simulink model "Optimal_lqr"  (R2018b)
settings: Solver=VariableStepAuto  StartTime=0.0  StopTime=10  RelTol=1e-3
InitFcn:
  | % NOTE: If using VoltPAQ-X1, make sure both Gain switches are set to 3.
  | K_AMP = 3;
  | % Maximum Output Voltage (V): YAW limited to 15 V. PITCH limited to 24 V.
  | VMAX_AMP_P = 24;
  | VMAX_AMP_Y = 15;
  | % Initial Angle of Pitch (rad)
  | theta_0 = -40.5*pi/180;
  | 
  | g = 9.81;
  | 
  | % Pitch and Yaw Motor Armature Resistance (Ohm)
  | R_m_p = 0.83;
  | R_m_y = 1.60;
  | 
  | % Pitch and Yaw Motor Current-Torque Constant (N.m/A)
  | K_t_p = 0.0182;
  | K_t_y = 0.0109;
  | 
  | % Pitch and Yaw Motor Voltage-Torque Constant (N.m/V)
  | K_yp = K_t_p / R_m_p;
  | K_py = K_t_y / R_m_y;
  | 
  | % Pitch and Yaw Viscous Damping Constant (N.m.s/rad)
  | B_p = 0.8;  % tuned while running simulation and experiment in parallel
  | B_y = 0.318; % identified as described in manual
  | 
  | % Mass of the Helicopter (kg)
  | m_heli = 1.3872;
  | 
  | % Mass of the Helicopter with Yoke (kg)
  | m_heli_case = 1.421;
  | 
  | % Distance from Pitch Pivot to Pitch/Front Motor and Yaw/Back Motor(m)
  | r_p = 7.75*0.0254;
  | r_y = (6+5/8)*0.0254;
  | 
  | % Pitch and Yaw Propeller Force-Thrust Constant found Experimentally (N/V)
  | K_f_p = 5*0.2074;
  | K_f_y = 3*0.1426;
  | 
  | % Pitch and Yaw Propeller Torque-Thrust Constant found Experimentally (N.m/V)
  | K_pp = K_f_p * r_p;
  | K_yy = K_f_y * r_y;
  | 
  | % Mass of Pitch/Front Motor and Yaw/Back Motor (kg)
  | m_motor_p = 0.292;
  | m_motor_y = 0.128;
  | 
  | % Mass of Pitch/Front and Yaw/Back Guard + Propeller(kg)
  | m_shield = 0.143 + 0.024;
  | 
  | % Total Mass of Pitch and Yaw Motor/Shield Assemblies (kg)
  | m_props = ( m_motor_p + m_motor_y + 2 * m_shield );
  | 
  | % Mass of Helicopter Body moving about Pitch Axis (kg)
  | m_body_p = m_heli - m_props;
  | 
  | % Mass of Helicopter Body moving about Yaw Axis (kg)
  | m_body_y = m_heli_case - m_props;
  | 
  | % Mass of Metal Shaft Moving about Yaw Axis (kg)
  | m_shaft = 0.151;
  | 
  | % Total Length of Helicopter Body (m)
  | L_body = 19*0.0254;
  | 
  | % Helicopter Center of Mass from Pivot along Pitch Axis (m)
  | l_cm = ( (m_motor_p + m_shield ) * r_p +  (m_motor_y + m_shield ) * r_y ) / ( m_props ) ;
  | 
  | % Length of Metal Shaft Moving about Yaw Axis through slip ring (m)
  | L_shaft = 11 * 0.0254;
  | 
  | % Pitch and Yaw Motor Rotor Moment of Inertia (kg.m^2)
  | J_m_p = 1.91e-6; %1.7070e-5;
  | J_m_y = 1.374e-4; %1.4471e-5;
  | 
  | % Moment of Inertia of Helicopter Body about its CM (kg.m^2)
  | J_body_p = m_body_p * L_body^2 / 12;
  | J_body_y = m_body_y * L_body^2 / 12;
  | 
  | % Moment of Inertia of Metal Shaft about Yaw Axis (kg.m^2)
  | J_shaft = m_shaft * L_shaft^2 / 3; %;0.0851;
  | 
  | % Moment of Inertia of Pitch Motor + Guard Assembly about Pivot (kg.m^2)
  | J_p = ( m_motor_p + m_shield ) * r_p^2;
  | 
  | % Moment of Inertia of Yaw Motor + Guard Assembly about Pivot (kg.m^2)
  | J_y = ( m_motor_y + m_shield ) * r_y^2;
  | 
  | % Equivalent Moment of Inertia about Pitch and Yaw Axis (kg.m^2)
  | J_eq_p = J_m_p + J_body_p + J_p + J_y;
  | J_eq_y = J_m_y + J_body_y + J_p + J_y + J_shaft;
  | 
  | 
  | %BESSEL wn=4
  | Kbes=[     68.5119  -25.1203    5.3421   -3.6881
  |    63.1652  188.4894    0.7783   19.4789];
  | 
  | xd=-20;
libraries: simulink x1
settings Model: Creator=rezan  LastModifiedBy=rezan
settings DataIOCC: ReturnWorkspaceOutputs=on
settings DebuggingCC: UnconnectedInputMsg=none  UnconnectedOutputMsg=none  UnconnectedLineMsg=none  SFMachineParentedDataDiag=error

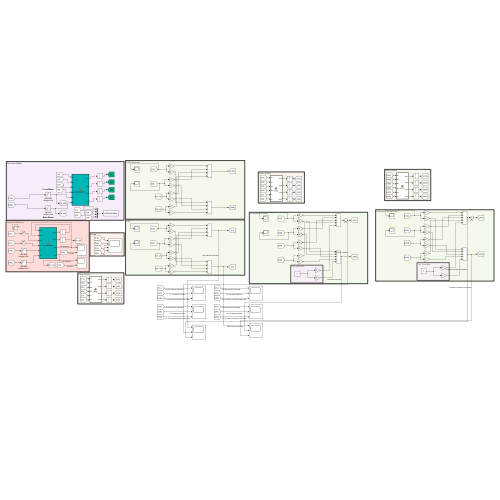
[thumbnail: Simulink's stored preview of the top-level diagram]
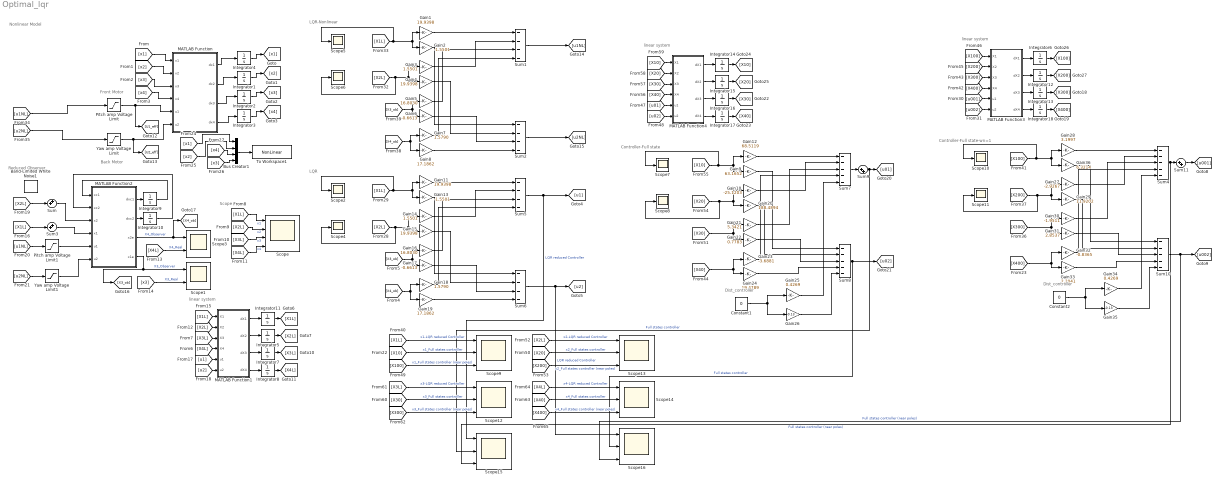
== system Optimal_lqr ==
  note: linear system
  note: Front Motor
  note: Back Motor
  note: Nonlinear Model
  note: Scope
  note: LQR
  note: Reduced Observer
  note: LQR-Nonlinear
  note: Dist_controller
  note: Controller-Full state
  note: linear system
  note: Dist_controller
  note: Controller-Full state-wn=1
  note: linear system
  Band-Limited White Noise1 : simulink/Sources/Band-Limited White Noise  Cov=[0.01]  Ts=0.1  seed=[23341]
  Bus Creator1 : BusCreator  Inputs=4
  Constant1 : Constant  Value=0
  Constant2 : Constant  Value=0
  Gain{1,4,11,15} (4 alike) : Gain  Gain=19.9398
  Gain10 : Gain  Gain=-25.1203
  Gain12 : Gain  Gain=68.5119
  Gain13 : Gain  Gain=-1.5501
  Gain14 : Gain  Gain=1.5501
  Gain16 : Gain  Gain=16.8030
  Gain17 : Gain  Gain=-0.6613
  Gain18 : Gain  Gain=1.5790
  Gain19 : Gain  Gain=17.1862
  Gain2 : Gain  Gain=-1.5501
  Gain20 : Gain  Gain=188.4894
  Gain21 : Gain  Gain=5.3421
  Gain22 : Gain  Gain=0.7783
  Gain23 : Gain  Gain=-3.6881
  Gain24 : Gain  Gain=19.4789
  Gain25 : Gain  Gain=0.4269
  Gain26 : Gain  Gain=-0.13
  Gain27 : Gain  Gain=-2.9267
  Gain28 : Gain  Gain=3.1997
  Gain29 : Gain  Gain=11.9202
  Gain3 : Gain  Gain=1.5501
  Gain30 : Gain  Gain=-1.9511
  Gain31 : Gain  Gain=2.8537
  Gain32 : Gain  Gain=-0.8365
  Gain33 : Gain  Gain=2.3041
  Gain34 : Gain  Gain=0.4269
  Gain35 : Gain  Gain=-0.13
  Gain36 : Gain  Gain=6.3214
  Gain5 : Gain  Gain=16.8030
  Gain6 : Gain  Gain=-0.6613
  Gain7 : Gain  Gain=1.5790
  Gain8 : Gain  Gain=17.1862
  Gain9 : Gain  Gain=63.1652
  Integrator{1,5,12,15} (4 alike) : Integrator  InitialCondition=10*pi/180
  Integrator{2..3,8..10,17..18} (7 alike) : Integrator
  Integrator{4,6,11,14} (4 alike) : Integrator  UpperSaturationLimit=40.5*pi/180  LowerSaturationLimit=-40.5*pi/180
  Integrator13 : Integrator  InitialCondition=10
  Integrator16 : Integrator  InitialCondition=10
  Integrator7 : Integrator  InitialCondition=10
  MATLAB Function : MATLAB Function  TreatAsAtomicUnit=on
  MATLAB Function1 : MATLAB Function  TreatAsAtomicUnit=on
  MATLAB Function2 : MATLAB Function  TreatAsAtomicUnit=on
  MATLAB Function3 : MATLAB Function  TreatAsAtomicUnit=on
  MATLAB Function4 : MATLAB Function  TreatAsAtomicUnit=on
  Pitch amp Voltage Limit : Saturate  UpperLimit=VMAX_AMP_P  LowerLimit=- VMAX_AMP_P
  Pitch amp Voltage Limit1 : Saturate  UpperLimit=VMAX_AMP_P  LowerLimit=- VMAX_AMP_P
  Scope : Scope  NumInputPorts=4
  Scope1 : Scope  NumInputPorts=2
  Scope{2,4..8,10..11} (8 alike) : Scope
  Scope{9,12..16} (6 alike) : Scope  NumInputPorts=3
  Scope3 : Scope  NumInputPorts=2
  Sum : Sum  Inputs=++|
  Sum{1..2,5..6} (4 alike) : Sum  Inputs=----
  Sum{4,7..8,10} (4 alike) : Sum  Inputs=-----
  Sum11 : Sum  Inputs=|++
  Sum3 : Sum  Inputs=++|
  Sum9 : Sum  Inputs=|++
  To Workspace1 : ToWorkspace  VariableName=NonLinear  SampleTime=-1
  Yaw amp Voltage Limit : Saturate  UpperLimit=VMAX_AMP_Y  LowerLimit=- VMAX_AMP_Y
  Yaw amp Voltage Limit1 : Saturate  UpperLimit=VMAX_AMP_Y  LowerLimit=- VMAX_AMP_Y
  wires:
  MATLAB Function/2(dx2) -> Integrator1/1
  [X1L] -> Gain13/1, Gain11/1, Scope2/1
  Gain11/1 -> Sum5/1
  Yaw amp Voltage Limit1/1 -> MATLAB Function2/6(u2)
  [X1L] -> Scope/1  "x1"
  Integrator2/1 -> [x3]
  [X2L] -> Gain15/1, Gain14/1, Scope4/1
  Integrator4/1 -> [x1]
  MATLAB Function/3(dx3) -> Integrator2/1
  MATLAB Function/1(dx1) -> Integrator4/1
  [x1] -> MATLAB Function/1(x1)
  [x1] -> Bus Creator1/1
  [x2] -> Bus Creator1/2
  [x3] -> MATLAB Function/3(x3)
  [x4] -> MATLAB Function/4(x4)
  [x3] -> Bus Creator1/4
  Integrator3/1 -> [x4]
  Integrator9/1 -> MATLAB Function2/1(xc1)
  Gain16/1 -> Sum5/3
  Bus Creator1/1 -> To Workspace1/1
  Integrator1/1 -> [x2]
  [X4L] -> Scope3/2  "X4_Real"
  MATLAB Function2/1(dxc1) -> Integrator9/1
  [u2NL] -> Yaw amp Voltage Limit1/1
  [x3] -> Scope1/2  "X3_Real"
  Yaw amp Voltage Limit/1 -> [U2_eff], MATLAB Function/6(u2)
  MATLAB Function2/4(x1e) -> Scope1/1, [X3_ob]  "X3_Observer"
  Pitch amp Voltage Limit1/1 -> MATLAB Function2/5(u1)
  Gain18/1 -> Sum5/4
  Gain17/1 -> Sum6/3
  MATLAB Function2/3(x2e) -> [X4_ob], Scope3/1  "X4_Observer"
  Integrator10/1 -> MATLAB Function2/2(xc2)
  [u1NL] -> Pitch amp Voltage Limit1/1
  Gain19/1 -> Sum6/4
  MATLAB Function2/2(dxc2) -> Integrator10/1
  Pitch amp Voltage Limit/1 -> [U1_eff], MATLAB Function/5(u1)
  Gain14/1 -> Sum5/2
  Gain15/1 -> Sum6/2
  MATLAB Function/4(dx4) -> Integrator3/1
  Gain13/1 -> Sum6/1
  [x2] -> MATLAB Function/2(x2)
  [x4] -> Bus Creator1/3
  [X2L] -> Scope/2  "x2"
  [X3L] -> Scope/3  "x3"
  [X4L] -> Scope/4  "x4"
  [u1NL] -> Pitch amp Voltage Limit/1
  [u2NL] -> Yaw amp Voltage Limit/1
  MATLAB Function1/4(dX4) -> Integrator8/1
  MATLAB Function1/1(dX1) -> Integrator11/1
  MATLAB Function1/2(dX2) -> Integrator5/1
  MATLAB Function1/3(dX3) -> Integrator7/1
  Integrator11/1 -> [X1L]
  Integrator5/1 -> [X2L]
  Integrator8/1 -> [X4L]
  Integrator7/1 -> [X3L]
  [X4L] -> MATLAB Function1/4(X4)
  [X3L] -> MATLAB Function1/3(X3)
  [X2L] -> MATLAB Function1/2(X2)
  [X1L] -> MATLAB Function1/1(X1)
  [u1] -> MATLAB Function1/5(u1)
  [u2] -> MATLAB Function1/6(u2)
  [X3_ob] -> Gain17/1, Gain16/1
  [X4_ob] -> Gain19/1, Gain18/1
  Sum6/1 -> Scope16/1, [u2]  "LQR reduced Controller"
  Sum5/1 -> Scope15/1, [u1]  "LQR reduced Controller"
  Sum1/1 -> [u1NL]
  Sum2/1 -> [u2NL]
  [X4_ob] -> Gain7/1, Gain8/1
  [X3_ob] -> Gain5/1, Gain6/1
  Gain2/1 -> Sum2/1
  Gain4/1 -> Sum2/2
  Gain3/1 -> Sum1/2
  Gain8/1 -> Sum2/4
  Gain6/1 -> Sum2/3
  Gain7/1 -> Sum1/4
  Gain5/1 -> Sum1/3
  [X2L] -> Scope6/1, Gain3/1, Gain4/1
  Gain1/1 -> Sum1/1
  [X1L] -> Scope5/1, Gain1/1, Gain2/1
  [X2L] -> Sum/2
  [X1L] -> Sum3/2
  Sum3/1 -> MATLAB Function2/4(x1)
  Sum/1 -> MATLAB Function2/3(x2)
  [X30] -> Gain22/1, Gain21/1
  [X10] -> Gain12/1, Gain9/1, Scope7/1
  Gain21/1 -> Sum7/3
  [X20] -> Gain20/1, Gain10/1, Scope8/1
  Gain26/1 -> Sum8/5
  Sum7/1 -> Sum9/1
  Sum9/1 -> Scope15/2, [u01]  "Full states controller"
  Gain24/1 -> Sum8/4
  Gain10/1 -> Sum7/2
  Gain23/1 -> Sum7/4
  Gain20/1 -> Sum8/2
  Sum8/1 -> Scope16/2, [u02]  "Full states controller"
  Gain12/1 -> Sum7/1
  [X40] -> Gain23/1, Gain24/1
  Gain9/1 -> Sum8/1
  Gain25/1 -> Sum7/5
  Gain22/1 -> Sum8/3
  Constant1/1 -> Gain25/1, Gain26/1
  [X1L] -> Scope9/1  "x1-LQR reduced Controller"
  [X10] -> Scope9/2  "x1_Full states controller"
  [u02] -> MATLAB Function4/6(u2)
  [u01] -> MATLAB Function4/5(u1)
  [X10] -> MATLAB Function4/1(X1)
  [X20] -> MATLAB Function4/2(X2)
  [X30] -> MATLAB Function4/3(X3)
  [X40] -> MATLAB Function4/4(X4)
  Integrator16/1 -> [X30]
  Integrator17/1 -> [X40]
  Integrator15/1 -> [X20]
  Integrator14/1 -> [X10]
  MATLAB Function4/3(dX3) -> Integrator16/1
  MATLAB Function4/2(dX2) -> Integrator15/1
  MATLAB Function4/1(dX1) -> Integrator14/1
  MATLAB Function4/4(dX4) -> Integrator17/1
  MATLAB Function3/4(dX4) -> Integrator18/1
  MATLAB Function3/1(dX1) -> Integrator6/1
  MATLAB Function3/2(dX2) -> Integrator12/1
  MATLAB Function3/3(dX3) -> Integrator13/1
  Integrator6/1 -> [X100]
  Integrator12/1 -> [X200]
  Integrator18/1 -> [X400]
  Integrator13/1 -> [X300]
  [X400] -> MATLAB Function3/4(X4)
  [X300] -> MATLAB Function3/3(X3)
  [X200] -> MATLAB Function3/2(X2)
  [X100] -> MATLAB Function3/1(X1)
  [u001] -> MATLAB Function3/5(u1)
  [u002] -> MATLAB Function3/6(u2)
  Constant2/1 -> Gain35/1, Gain34/1
  Gain31/1 -> Sum10/3
  Gain34/1 -> Sum4/5
  Gain36/1 -> Sum10/1
  [X400] -> Gain33/1, Gain32/1
  Gain28/1 -> Sum4/1
  Sum10/1 -> Scope16/3, [u002]  "Full states controller (near poles)"
  Gain29/1 -> Sum10/2
  Gain32/1 -> Sum4/4
  Gain27/1 -> Sum4/2
  Gain33/1 -> Sum10/4
  Sum11/1 -> [u001]
  Sum4/1 -> Scope15/3, Sum11/1  "Full states controller (near poles)"
  Gain35/1 -> Sum10/5
  [X200] -> Scope11/1, Gain27/1, Gain29/1
  Gain30/1 -> Sum4/3
  [X100] -> Scope10/1, Gain36/1, Gain28/1
  [X300] -> Gain30/1, Gain31/1
  [X100] -> Scope9/3  "x1_Full states controller (near poles)"
  [X200] -> Scope13/3  "x2_Full states controller (near poles)"
  [X20] -> Scope13/2  "x2_Full states controller"
  [X2L] -> Scope13/1  "x2-LQR reduced Controller"
  [X3L] -> Scope12/1  "x3-LQR reduced Controller"
  [X30] -> Scope12/2  "x3_Full states controller"
  [X300] -> Scope12/3  "x3_Full states controller (near poles)"
  [X400] -> Scope14/3  "x4_Full states controller (near poles)"
  [X40] -> Scope14/2  "x4_Full states controller"
  [X4L] -> Scope14/1  "x4-LQR reduced Controller"

== matlab function Optimal_lqr/MATLAB Function1 ==
  data: X1 input; dX1 output; X2 input; X3 input; X4 input; u1 input; dX2 output; dX3 output; dX4 output; u2 input
function [dX1,dX2,dX3,dX4] = Linear(X1,X2,X3,X4,u1,u2)
%#codegen

A=[      0         0    1.0000         0
         0         0         0    1.0000
         0         0   -9.2751         0
         0         0         0   -3.4955];
     
B=[      0         0
         0         0
    2.3667    0.0790
    0.2410    0.7913];

X = [X1;X2;X3;X4];
U=[u1,u2].';
dX = A*X+B*U;
dX1 = dX(1);
dX2 = dX(2);
dX3 = dX(3);
dX4 = dX(4);

== matlab function Optimal_lqr/MATLAB Function2 ==
  data: xc1 input; xc2 input; x2 input; x1 input; u1 input; dxc1 output; dxc2 output; x2e output; x1e output; u2 input
function [dxc1,dxc2,x2e,x1e] = Re_Observer(xc1,xc2,x2,x1,u1,u2)

A=[      0         0    1.0000         0
         0         0         0    1.0000
         0         0   -9.2751         0
         0         0         0   -3.4955];
     
B=[      0         0
         0         0
    2.3667    0.0790
    0.2410    0.7913];
C=[  1     0     0     0
     0     1     0     0];

 D=[  0     0
     0     0];

 
C = eye(2,4);
Aee = A(3:4,3:4);
Aes = A(3:4,1:2);
Ase = A(1:2,3:4);
Ass = A(1:2,1:2);

Be = B(3:4,1);
Bs = B(1:2,1);
u=[u1 u2];
Cs = C(1:2,1:2);
L = [   40.7249         0
         0   56.5045];

% 
%  L=  [-4.2751         0
%          0    2.5045];


xc = [xc1;xc2];
y = [x1;x2];
xs = [x1;x2];
dxc = (Aee-L*Cs*Ase)*(xc+L*y)+(Aes*inv(Cs)-L*Cs*Ass*inv(Cs))*y+(Be-L*Cs*Bs)*u;
dxc1 = dxc(1);
dxc2 = dxc(2);
Xe = xc+L*y;
x1e = Xe(1);
x2e = Xe(2);

== matlab function Optimal_lqr/MATLAB Function3 ==
  data: X1 input; dX1 output; X2 input; X3 input; X4 input; u1 input; dX2 output; dX3 output; dX4 output; u2 input
function [dX1,dX2,dX3,dX4] = Linear(X1,X2,X3,X4,u1,u2)
%#codegen

A=[      0         0    1.0000         0
         0         0         0    1.0000
         0         0   -9.2751         0
         0         0         0   -3.4955];
     
B=[      0         0
         0         0
    2.3667    0.0790
    0.2410    0.7913];

X = [X1;X2;X3;X4];
U=[u1,u2].';
dX = A*X+B*U;
dX1 = dX(1);
dX2 = dX(2);
dX3 = dX(3);
dX4 = dX(4);

== matlab function Optimal_lqr/MATLAB Function4 ==
  data: X1 input; dX1 output; X2 input; X3 input; X4 input; u1 input; dX2 output; dX3 output; dX4 output; u2 input
function [dX1,dX2,dX3,dX4] = Linear(X1,X2,X3,X4,u1,u2)
%#codegen

A=[      0         0    1.0000         0
         0         0         0    1.0000
         0         0   -9.2751         0
         0         0         0   -3.4955];
     
B=[      0         0
         0         0
    2.3667    0.0790
    0.2410    0.7913];

X = [X1;X2;X3;X4];
U=[u1,u2].';
dX = A*X+B*U;
dX1 = dX(1);
dX2 = dX(2);
dX3 = dX(3);
dX4 = dX(4);

== matlab function Optimal_lqr/MATLAB Function ==
  data: x1 input; x2 input; x3 input; x4 input; u1 input; dx1 output; u2 input; dx2 output; dx3 output; dx4 output
function [dx1,dx2,dx3,dx4]= NonlinearFunc(x1,x2,x3,x4,u1,u2)
%% Initial Conditions
% Gravitational Constant (m/s^2)
g = 9.81;

% Pitch and Yaw Motor Armature Resistance (Ohm)
R_m_p = 0.83;
R_m_y = 1.60;

% Pitch and Yaw Motor Current-Torque Constant (N.m/A)
K_t_p = 0.0182;
K_t_y = 0.0109;

% Pitch and Yaw Motor Voltage-Torque Constant (N.m/V)
K_yp = K_t_p / R_m_p;
K_py = K_t_y / R_m_y;

% Pitch and Yaw Viscous Damping Constant (N.m.s/rad)
B_p = 0.8;  % tuned while running simulation and experiment in parallel
B_y = 0.318; % identified as described in manual 

% Mass of the Helicopter (kg)
m_heli = 1.3872;

% Mass of the Helicopter with Yoke (kg)
m_heli_case = 1.421;

% Distance from Pitch Pivot to Pitch/Front Motor and Yaw/Back Motor(m)
r_p = 7.75*0.0254;
r_y = (6+5/8)*0.0254;

% Pitch and Yaw Propeller Force-Thrust Constant found Experimentally (N/V)
K_f_p = 5*0.2074;
K_f_y = 3*0.1426;

% Pitch and Yaw Propeller Torque-Thrust Constant found Experimentally (N.m/V)
K_pp = K_f_p * r_p;
K_yy = K_f_y * r_y;

% Mass of Pitch/Front Motor and Yaw/Back Motor (kg)
m_motor_p = 0.292;
m_motor_y = 0.128;

% Mass of Pitch/Front and Yaw/Back Guard + Propeller(kg)
m_shield = 0.143 + 0.024;

% Total Mass of Pitch and Yaw Motor/Shield Assemblies (kg)
m_props = ( m_motor_p + m_motor_y + 2 * m_shield );

% Mass of Helicopter Body moving about Pitch Axis (kg)
m_body_p = m_heli - m_props; 

% Mass of Helicopter Body moving about Yaw Axis (kg)
m_body_y = m_heli_case - m_props; 

% Mass of Metal Shaft Moving about Yaw Axis (kg)
m_shaft = 0.151;

% Total Length of Helicopter Body (m)
L_body = 19*0.0254;

% Helicopter Center of Mass from Pivot along Pitch Axis (m)
l_cm = ( (m_motor_p + m_shield ) * r_p +  (m_motor_y + m_shield ) * r_y ) / ( m_props ) ;

% Length of Metal Shaft Moving about Yaw Axis through slip ring (m)
L_shaft = 11 * 0.0254;

% Pitch and Yaw Motor Rotor Moment of Inertia (kg.m^2)
J_m_p = 1.91e-6; %1.7070e-5;
J_m_y = 1.374e-4; %1.4471e-5;

% Moment of Inertia of Helicopter Body about its CM (kg.m^2)
J_body_p = m_body_p * L_body^2 / 12;
J_body_y = m_body_y * L_body^2 / 12;

% Moment of Inertia of Metal Shaft about Yaw Axis (kg.m^2)
J_shaft = m_shaft * L_shaft^2 / 3; %;0.0851;

% Moment of Inertia of Pitch Motor + Guard Assembly about Pivot (kg.m^2)
J_p = ( m_motor_p + m_shield ) * r_p^2;

% Moment of Inertia of Yaw Motor + Guard Assembly about Pivot (kg.m^2)
J_y = ( m_motor_y + m_shield ) * r_y^2;

% Equivalent Moment of Inertia about Pitch and Yaw Axis (kg.m^2)
J_eq_p = J_m_p + J_body_p + J_p + J_y;
J_eq_y = J_m_y + J_body_y + J_p + J_y + J_shaft;
%%
%%
xd=0
 dx1=x3;
dx2=x4;
dx3=(1/(J_eq_p +m_heli*l_cm^2))*((K_pp*u1+K_py*u2)-(B_p*x3+m_heli*l_cm^2*x4^2*sin(x1)*cos(x1)+m_heli*g*l_cm*cos(x1)));
dx3=dx3+xd;
dx4=1/(J_eq_y + m_heli *l_cm^2* (cos(x1))^2 )*((K_yp*u1 )+(K_yy*u2 ))+(-B_y*x4+2*m_heli*l_cm^2*x4*x3*sin(x1)*cos(x1))/(J_eq_p+ m_heli * l_cm^2 * (cos(x1))^2);
